simulink model "gyro"  (R2020b)
settings: Solver=VariableStepAuto  StartTime=0.0  StopTime=10.0  RelTol=1e-3
model mask{g_sf_cc=[1, 0, 0; 0, 1, 0; 0, 0, 1], g_sen=[0 0 0], g_bias=[0 0 0], g_noise=[0 0 0], g_sath=[inf inf inf], g_satl=[-inf -inf -inf], sample_rate=100}
  mask prompts: g_sf_cc "Scale factors and cross coupling:"; g_sen "G-sensitivity [rad/s per m/s/s]:"; g_bias "Bias [rad/s]:"; g_noise "Noise [rad/s]:"; g_sath "Upper limits [rad/s]:"; g_satl "Lower limits [rad/s]:"; sample_rate "Sample Rate [Hz]:"
model workspace (MAT data in the model file):
  g_bias = Simulink.Parameter
  g_bias.Value = [0 0 0]
  g_bias.DataType = 'auto'
  g_bias.Dimensions = [1 3]
  g_noise = Simulink.Parameter
  g_noise.Value = [0 0 0]
  g_noise.DataType = 'auto'
  g_noise.Dimensions = [1 3]
  g_sath = Simulink.Parameter
  g_sath.Value = [Inf Inf Inf]
  g_sath.DataType = 'auto'
  g_sath.Dimensions = [1 3]
  g_satl = Simulink.Parameter
  g_satl.Value = [-Inf -Inf -Inf]
  g_satl.DataType = 'auto'
  g_satl.Dimensions = [1 3]
  g_sen = Simulink.Parameter
  g_sen.Value = [0 0 0]
  g_sen.DataType = 'auto'
  g_sen.Dimensions = [1 3]
  g_sf_cc = Simulink.Parameter
  g_sf_cc.Value = [1  0  0; 0  1  0; 0  0  1]
  g_sf_cc.DataType = 'auto'
  g_sf_cc.Dimensions = [3 3]
  sample_rate = Simulink.Parameter
  sample_rate.Value = 100
  sample_rate.DataType = 'auto'
  sample_rate.Dimensions = [1 1]
libraries: simulink x1
settings Model: ParameterArgumentNames=g_bias,g_noise,g_sath,g_satl,g_sen,g_sf_cc,sample_rate  OrderedModelArguments=off  Creator=brian  LastModifiedBy=brian

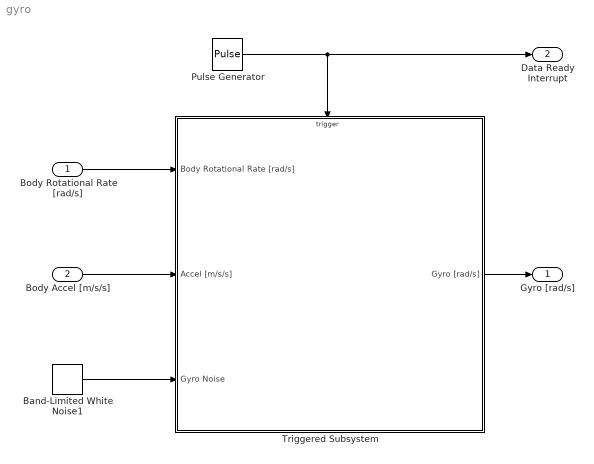
== system gyro ==
  Body Rotational Rate [rad/s] : Inport
  Body Accel [m/s/s] : Inport  Port=2
  Band-Limited White Noise1 : simulink/Sources/Band-Limited White Noise  Cov=g_noise  Ts=0.1  seed=[23341]
  Pulse Generator : DiscretePulseGenerator  PulseType=Time based  Period=1/sample_rate  PulseWidth=5
  Triggered Subsystem : Subsystem  TreatAsAtomicUnit=on
  Gyro [rad/s] : Outport
  Data Ready Interrupt : Outport  Port=2
  wires:
  Body Accel [m/s/s]/1 -> Triggered Subsystem/2(Accel [m/s/s])
  Body Rotational Rate [rad/s]/1 -> Triggered Subsystem/1(Body Rotational Rate [rad/s])
  Triggered Subsystem/1(Gyro [rad/s]) -> Gyro [rad/s]/1
  Pulse Generator/1 -> Data Ready Interrupt/1, Triggered Subsystem/Trigger
  Band-Limited White Noise1/1 -> Triggered Subsystem/3(Gyro Noise)

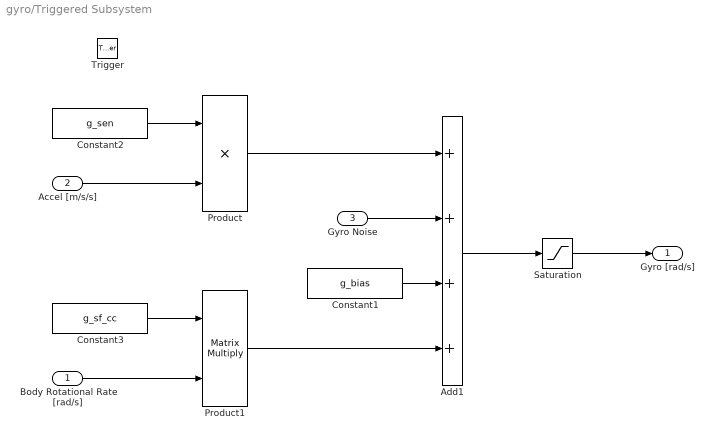
== system gyro/Triggered Subsystem ==
  Body Rotational Rate [rad/s] : Inport  PortDimensions=3
  Accel [m/s/s] : Inport  Port=2  PortDimensions=3
  Gyro Noise : Inport  Port=3  PortDimensions=3
  Trigger : TriggerPort  VariantControl=Variant
  Add1 : Sum  Inputs=++++
  Constant1 : Constant  Value=g_bias
  Constant2 : Constant  Value=g_sen
  Constant3 : Constant  Value=g_sf_cc
  Product : Product
  Product1 : Product  Multiplication=Matrix(*)
  Saturation : Saturate  UpperLimit=g_sath  LowerLimit=g_satl
  Gyro [rad/s] : Outport  PortDimensions=3
  wires:
  Product1/1 -> Add1/4
  Constant1/1 -> Add1/3
  Gyro Noise/1 -> Add1/2
  Product/1 -> Add1/1
  Add1/1 -> Saturation/1
  Accel [m/s/s]/1 -> Product/2
  Constant2/1 -> Product/1
  Body Rotational Rate [rad/s]/1 -> Product1/2
  Constant3/1 -> Product1/1
  Saturation/1 -> Gyro [rad/s]/1
